simulink model "TV_2021"  (R2017b)
settings: Solver=VariableStepAuto  StartTime=0.0  StopTime=10.0  RelTol=1e-3
undefined symbols (not defined in the file): sigbuilder_block
libraries: simulink x6
(part 8 of 13)

== system TV_2021/Vehicle Dynamics Control 2018/Steering TV 2017 with TC/Constraints/current_limitation1/constants_saturator ==
  note: Saturamos con unos
      | valores máximos
      | preestablecidos
  allowed_current [%] : Inport
  max_discharge_current : Inport  Port=2
  max_regen_current : Inport  Port=3
  Constant : Constant  Value=0
  Gain2 : Gain  Gain=-1
  Saturation Dynamic : simulink/Discontinuities/Saturation Dynamic  OutMin=[]  OutMax=[]  OutDataTypeStr=Inherit: Same as second input  OutDataType=fixdt(1, 16)  OutScaling=2^-10  DoSatur=off
  Saturation Dynamic1 : simulink/Discontinuities/Saturation Dynamic  OutMin=[]  OutMax=[]  OutDataTypeStr=Inherit: Same as second input  OutDataType=fixdt(1, 16)  OutScaling=2^-10  DoSatur=off
  limited_discharge_actual : Outport  VectorParamsAs1DForOutWhenUnconnected=on
  limited_regen_actual : Outport  Port=2  VectorParamsAs1DForOutWhenUnconnected=on
  wires:
  max_regen_current/1 -> Saturation Dynamic1/1
  Constant/1 -> Saturation Dynamic/3, Saturation Dynamic1/3
  Gain2/1 -> Saturation Dynamic1/2
  Saturation Dynamic1/1 -> limited_regen_actual/1
  allowed_current [%]/1 -> Saturation Dynamic/2, Gain2/1
  Saturation Dynamic/1 -> limited_discharge_actual/1
  max_discharge_current/1 -> Saturation Dynamic/1

== system TV_2021/Vehicle Dynamics Control 2018/Steering TV 2017 with TC/Constraints/current_limitation1/temperature_rise_limitator ==
  note: initial_limitation es una constante para la reducción inicial (de 0 a 1, más bajo significa que cambia
      | menos, más alto la limitación
      | inicial es más bestia).
  note: saturamos de 1 a 0 por si acaso
  note: magia chunga para
      | que los números cuadren
  note: Se limita la corriente en proporción
      | al ratio entre la temperatura actual y 50ºC
  note: output 0 si está por
      | debajo de 50ºC, 1 si está
      | por encima
  max_cell_temp : Inport
  initial_limitation : Inport  Port=2
  Add1 : Sum  Inputs=-+
  Add2 : Sum  Inputs=-++
  Add3 : Sum  Inputs=+-
  Constant1 : Constant  Value=55
  Constant2 : Constant  Value=5
  Constant3 : Constant
  Divide : Product  Inputs=*/
  Product4 : Product
  Saturation1 : Saturate  UpperLimit=1  LowerLimit=0
  Scope2 : Scope
  Scope4 : Scope
  Temp higher than 50 : simulink/Logic and Bit Operations/Compare To Constant  relop=>=  const=50  OutDataTypeStr=boolean  ZeroCross=off
  allowed_current : Outport  VectorParamsAs1DForOutWhenUnconnected=on
  wires:
  Divide/1 -> Add3/1
  Constant3/1 -> Add2/3
  Constant1/1 -> Divide/1
  max_cell_temp/1 -> Add1/2, Scope4/1, Temp higher than 50/1
  Temp higher than 50/1 -> Add2/1, Product4/2
  Constant2/1 -> Add1/1
  Product4/1 -> Add2/2
  Add2/1 -> Scope2/1, Saturation1/1
  Add3/1 -> Product4/1
  Add1/1 -> Divide/2
  Saturation1/1 -> allowed_current/1
  initial_limitation/1 -> Add3/2

== system TV_2021/Vehicle Dynamics Control 2018/Steering TV 2017 with TC/Optimization SKF & CKF/Subsystem /CKF ==
  Derivative : Inport
  CKF_Initial : Inport  Port=2
  "CKF_prev " : Inport  Port=3
  Cte_CKF : Inport  Port=4
  Action Port : ActionPort
  If1 : If  IfExpression=u1 >= 900  ElseIfExpressions=u1 < 900  ShowElse=off
  Merge : Merge
  No spin : Subsystem  TreatAsAtomicUnit=on
  Saturation : Saturate  UpperLimit=1  LowerLimit=0.3
  "Spin " : Subsystem  TreatAsAtomicUnit=on
  "CKF_act " : Outport
  wires:
  Merge/1 -> Saturation/1
  "CKF_prev "/1 -> "Spin "/1(CKF_prev), No spin/2(CKF_prev)
  If1/1 -> "Spin "/Action
  Cte_CKF/1 -> "Spin "/3(Cte_CKF)
  "Spin "/1("CKF_act1 ") -> Merge/2
  Saturation/1 -> "CKF_act "/1
  CKF_Initial/1 -> "Spin "/2("CKF_Initial "), No spin/1(CKF_Initial)
  If1/2 -> No spin/Action
  No spin/1(CKF_act0) -> Merge/1
  Derivative/1 -> If1/1

== system TV_2021/Vehicle Dynamics Control 2018/Steering TV 2017 with TC/Optimization SKF & CKF/Subsystem /SKF ==
  Derivative : Inport
  "SKF_Initial " : Inport  Port=2
  SKF_prev : Inport  Port=3
  Cte_SKF : Inport  Port=4
  Action Port : ActionPort
  Display : Display
  Display1 : Display
  If : If  IfExpression=u1 >=900  ElseIfExpressions=u1 < 900  ShowElse=off
  Merge : Merge
  No spin : Subsystem  TreatAsAtomicUnit=on
  Saturation : Saturate  UpperLimit=1  LowerLimit=0.3
  Spin : Subsystem  TreatAsAtomicUnit=on
  SKF_act : Outport
  wires:
  Merge/1 -> Saturation/1
  Spin/1(SKF_act1) -> Merge/2
  "SKF_Initial "/1 -> Spin/1(SKF_Initial), No spin/1(SKF_Initial)
  No spin/1(SKF_act0) -> Merge/1
  If/2 -> No spin/Action
  SKF_prev/1 -> Display/1, Spin/2(SKF_prev), No spin/2(SKF_prev)
  Cte_SKF/1 -> Spin/3(Cte_SKF)
  Saturation/1 -> Display1/1, SKF_act/1
  If/1 -> Spin/Action
  Derivative/1 -> If/1

== system TV_2021/Vehicle Dynamics Control 2018/VDC 2018 Complete/Constraints/Acelerating and braking without Regenerative/Control de Potencia  ==
  Tq_RR : Inport
  Tq_RL : Inport  Port=2
  ReductionCte : Inport  Port=3
  Action Port : ActionPort
  Add : Sum  Inputs=+-
  Add1 : Sum  Inputs=+-
  Constant : Constant  Value=0
  Constant1 : Constant
  Product : Product
  Product1 : Product
  Tq_RR_out : Outport
  Tq_RL_out : Outport  Port=2
  Flag_Temperature : Outport  Port=3
  Flag_Power : Outport  Port=4
  wires:
  Tq_RR/1 -> Product/1, Add/1
  Tq_RL/1 -> Product1/1, Add1/1
  ReductionCte/1 -> Product/2, Product1/2
  Product1/1 -> Add1/2
  Product/1 -> Add/2
  Add1/1 -> Tq_RL_out/1
  Add/1 -> Tq_RR_out/1
  Constant1/1 -> Flag_Power/1
  Constant/1 -> Flag_Temperature/1

== system TV_2021/Vehicle Dynamics Control 2018/VDC 2018 Complete/Constraints/Acelerating and braking without Regenerative/Control de Temperatura ==
  Tq_RR : Inport
  Tq_RL : Inport  Port=2
  ReductionCte : Inport  Port=3
  Action Port : ActionPort
  Add : Sum  Inputs=+-
  Add1 : Sum  Inputs=+-
  Constant : Constant
  Constant1 : Constant  Value=0
  Product : Product
  Product1 : Product
  Tq_RR_out : Outport
  Tq_RL_out : Outport  Port=2
  Flag_Temperature : Outport  Port=3
  Flag_Power : Outport  Port=4
  wires:
  Add/1 -> Tq_RR_out/1
  Add1/1 -> Tq_RL_out/1
  Product/1 -> Add/2
  Product1/1 -> Add1/2
  ReductionCte/1 -> Product1/2, Product/2
  Tq_RL/1 -> Add1/1, Product1/1
  Tq_RR/1 -> Add/1, Product/1
  Constant1/1 -> Flag_Power/1
  Constant/1 -> Flag_Temperature/1

== system TV_2021/Vehicle Dynamics Control 2018/VDC 2018 Complete/Constraints/Acelerating and braking without Regenerative/If Action 1 ==
  Trans_max_dynamic : Inport
  Action Port : ActionPort
  Trans_limit : Outport
  wires:
  Trans_max_dynamic/1 -> Trans_limit/1

== system TV_2021/Vehicle Dynamics Control 2018/VDC 2018 Complete/Constraints/Acelerating and braking without Regenerative/If Action 2 ==
  "Trans_max_static " : Inport
  Action Port : ActionPort
  Trans_limit : Outport
  wires:
  "Trans_max_static "/1 -> Trans_limit/1

== system TV_2021/Vehicle Dynamics Control 2018/VDC 2018 Complete/Constraints/Acelerating and braking without Regenerative/Momentum Z scaled ==
  Tq_RR_Lim : Inport
  Tq_RL_Lim : Inport  Port=2
  Tq_RR_wc : Inport  Port=3
  Tq_RL_wc : Inport  Port=4
  Tq_diff : Inport  Port=5
  Display : Display
  Display1 : Display
  MATLAB Function : MATLAB Function  TreatAsAtomicUnit=on
  TQ_RR : Outport
  TQ_RL : Outport  Port=2
  wires:
  Tq_RL_Lim/1 -> MATLAB Function/2(tq_RL_lim)
  Tq_RR_Lim/1 -> MATLAB Function/1(tq_RR_lim)
  Tq_RR_wc/1 -> MATLAB Function/3(tq_RR_wc)
  Tq_RL_wc/1 -> MATLAB Function/4(tq_RL_wc)
  MATLAB Function/1(TQ_RR) -> Display/1, TQ_RR/1
  MATLAB Function/2(TQ_RL) -> Display1/1, TQ_RL/1
  Tq_diff/1 -> MATLAB Function/5(tq_diff)

== system TV_2021/Vehicle Dynamics Control 2018/VDC 2018 Complete/Constraints/Acelerating and braking without Regenerative/else ==
  Tq_RR : Inport
  Tq_RL : Inport  Port=2
  Action Port : ActionPort
  Constant : Constant  Value=0
  Constant1 : Constant  Value=0
  Tq_RR_out : Outport
  Tq_RL_out : Outport  Port=2
  Flag_Temperature : Outport  Port=3
  Flag_Power : Outport  Port=4
  wires:
  Tq_RR/1 -> Tq_RR_out/1
  Tq_RL/1 -> Tq_RL_out/1
  Constant1/1 -> Flag_Power/1
  Constant/1 -> Flag_Temperature/1

== system TV_2021/Vehicle Dynamics Control 2018/VDC 2018 Complete/Lateral Dynamics/Tire Longitudinal Force Difference/ Momentum_Z to Longitudinal Force Difference ==
  "\tMomentumZ [Nm]" : Inport
  RearTrackwidth [m] : Inport  Port=2
  Constant : Constant  Value=2
  Divide : Product  Inputs=*/
  Divide1 : Product  Inputs=*/
  Fx_diff [N] : Outport
  wires:
  Divide/1 -> Fx_diff [N]/1
  Divide1/1 -> Divide/2
  "\tMomentumZ [Nm]"/1 -> Divide/1
  Constant/1 -> Divide1/2
  RearTrackwidth [m]/1 -> Divide1/1

== system TV_2021/Vehicle Dynamics Control 2018/VDC 2018 Complete/Lateral Dynamics/Tire Longitudinal Force Difference/Momentum respect to Z-axis to correct the error ==
  Yaw_error_[º/s] : Inport
  Iz [kg/m^3] : Inport  Port=2
  Correction_Time [s] : Inport  Port=3
  Divide : Product  Inputs=*/
  Product : Product
  Momentum_Z [Nm] : Outport
  wires:
  Divide/1 -> Momentum_Z [Nm]/1
  Correction_Time [s]/1 -> Divide/2
  Product/1 -> Divide/1
  Yaw_error_[º/s]/1 -> Product/1
  Iz [kg/m^3]/1 -> Product/2

== system TV_2021/Vehicle Dynamics Control 2018/VDC 2018 Complete/Optimization SKF & CKF/Subsystem /CKF ==
  Derivative : Inport
  CKF_Initial : Inport  Port=2
  "CKF_prev " : Inport  Port=3
  Cte_CKF : Inport  Port=4
  Action Port : ActionPort
  If1 : If  IfExpression=u1 >= 900  ElseIfExpressions=u1 < 900  ShowElse=off
  Merge : Merge
  No spin : Subsystem  TreatAsAtomicUnit=on
  Saturation : Saturate  UpperLimit=1  LowerLimit=0.3
  "Spin " : Subsystem  TreatAsAtomicUnit=on
  "CKF_act " : Outport
  wires:
  Merge/1 -> Saturation/1
  "CKF_prev "/1 -> "Spin "/1(CKF_prev), No spin/2(CKF_prev)
  If1/1 -> "Spin "/Action
  Derivative/1 -> If1/1
  Cte_CKF/1 -> "Spin "/3(Cte_CKF)
  "Spin "/1("CKF_act1 ") -> Merge/2
  Saturation/1 -> "CKF_act "/1
  CKF_Initial/1 -> "Spin "/2("CKF_Initial "), No spin/1(CKF_Initial)
  If1/2 -> No spin/Action
  No spin/1(CKF_act0) -> Merge/1

== system TV_2021/Vehicle Dynamics Control 2018/VDC 2018 Complete/Optimization SKF & CKF/Subsystem /SKF ==
  Derivative : Inport
  "SKF_Initial " : Inport  Port=2
  SKF_prev : Inport  Port=3
  Cte_SKF : Inport  Port=4
  Action Port : ActionPort
  Display : Display
  If : If  IfExpression=u1 >=900  ElseIfExpressions=u1 < 900  ShowElse=off
  Merge : Merge
  No spin : Subsystem  TreatAsAtomicUnit=on
  Saturation : Saturate  UpperLimit=1  LowerLimit=0.3
  Spin : Subsystem  TreatAsAtomicUnit=on
  SKF_act : Outport
  wires:
  Merge/1 -> Saturation/1
  Derivative/1 -> If/1, Display/1
  Spin/1(SKF_act1) -> Merge/2
  "SKF_Initial "/1 -> Spin/1(SKF_Initial), No spin/1(SKF_Initial)
  No spin/1(SKF_act0) -> Merge/1
  If/2 -> No spin/Action
  SKF_prev/1 -> Spin/2(SKF_prev), No spin/2(SKF_prev)
  Cte_SKF/1 -> Spin/3(Cte_SKF)
  Saturation/1 -> SKF_act/1
  If/1 -> Spin/Action

== system TV_2021/Vehicle Dynamics Control 2018/VDC 2018 without Longitudinal/Constraints/Acelerating and braking without Regenerative/Control de Potencia 1 ==
  Tq_RR : Inport
  Tq_RL : Inport  Port=2
  ReductionCte : Inport  Port=3
  Action Port : ActionPort
  Add : Sum  Inputs=+-
  Add1 : Sum  Inputs=+-
  Product : Product
  Product1 : Product
  Tq_RR_out : Outport
  Tq_RL_out : Outport  Port=2
  wires:
  Tq_RR/1 -> Product/1, Add/1
  Tq_RL/1 -> Product1/1, Add1/1
  ReductionCte/1 -> Product/2, Product1/2
  Product1/1 -> Add1/2
  Product/1 -> Add/2
  Add1/1 -> Tq_RL_out/1
  Add/1 -> Tq_RR_out/1

== system TV_2021/Vehicle Dynamics Control 2018/VDC 2018 without Longitudinal/Constraints/Acelerating and braking without Regenerative/Control de Temperatura1 ==
  Tq_RR : Inport
  Tq_RL : Inport  Port=2
  ReductionCte : Inport  Port=3
  Action Port : ActionPort
  Add : Sum  Inputs=+-
  Add1 : Sum  Inputs=+-
  Product : Product
  Product1 : Product
  Tq_RR_out : Outport
  Tq_RL_out : Outport  Port=2
  wires:
  Product/1 -> Add/2
  Product1/1 -> Add1/2
  Add1/1 -> Tq_RL_out/1
  Tq_RR/1 -> Add/1, Product/1
  Tq_RL/1 -> Add1/1, Product1/1
  ReductionCte/1 -> Product1/2, Product/2
  Add/1 -> Tq_RR_out/1

== system TV_2021/Vehicle Dynamics Control 2018/VDC 2018 without Longitudinal/Constraints/Acelerating and braking without Regenerative/If Action 1 ==
  Trans_max_dynamic : Inport
  Action Port : ActionPort
  Trans_limit : Outport
  wires:
  Trans_max_dynamic/1 -> Trans_limit/1

== system TV_2021/Vehicle Dynamics Control 2018/VDC 2018 without Longitudinal/Constraints/Acelerating and braking without Regenerative/If Action 2 ==
  "Trans_max_static " : Inport
  Action Port : ActionPort
  Trans_limit : Outport
  wires:
  "Trans_max_static "/1 -> Trans_limit/1

== system TV_2021/Vehicle Dynamics Control 2018/VDC 2018 without Longitudinal/Constraints/Acelerating and braking without Regenerative/Momentum Z scaled ==
  Tq_RR_Lim : Inport
  Tq_RL_Lim : Inport  Port=2
  Tq_RR_wc : Inport  Port=3
  Tq_RL_wc : Inport  Port=4
  MATLAB Function : MATLAB Function  TreatAsAtomicUnit=on
  TQ_RR : Outport
  TQ_RL : Outport  Port=2
  wires:
  Tq_RL_Lim/1 -> MATLAB Function/2(tq_RL_lim)
  Tq_RR_Lim/1 -> MATLAB Function/1(tq_RR_lim)
  Tq_RR_wc/1 -> MATLAB Function/3(tq_RR_wc)
  Tq_RL_wc/1 -> MATLAB Function/4(tq_RL_wc)
  MATLAB Function/1(TQ_RR) -> TQ_RR/1
  MATLAB Function/2(TQ_RL) -> TQ_RL/1

== system TV_2021/Vehicle Dynamics Control 2018/VDC 2018 without Longitudinal/Constraints/Acelerating and braking without Regenerative/else1 ==
  Tq_RR : Inport
  Tq_RL : Inport  Port=2
  Action Port : ActionPort
  Tq_RR_out : Outport
  Tq_RL_out : Outport  Port=2
  wires:
  Tq_RR/1 -> Tq_RR_out/1
  Tq_RL/1 -> Tq_RL_out/1

== system TV_2021/Vehicle Dynamics Control 2018/VDC 2018 without Longitudinal/Optimization SKF & CKF/Subsystem /CKF ==
  Derivative : Inport
  CKF_Initial : Inport  Port=2
  "CKF_prev " : Inport  Port=3
  Cte_CKF : Inport  Port=4
  If1 : If  IfExpression=u1 >= 900  ElseIfExpressions=u1 < 900  ShowElse=off
  Merge : Merge
  No spin : Subsystem  TreatAsAtomicUnit=on
  Saturation : Saturate  UpperLimit=1  LowerLimit=0.3
  "Spin " : Subsystem  TreatAsAtomicUnit=on
  "CKF_act " : Outport
  wires:
  Merge/1 -> Saturation/1
  "CKF_prev "/1 -> "Spin "/1(CKF_prev), No spin/2(CKF_prev)
  Derivative/1 -> If1/1
  Cte_CKF/1 -> "Spin "/3(Cte_CKF)
  "Spin "/1("CKF_act1 ") -> Merge/2
  Saturation/1 -> "CKF_act "/1
  CKF_Initial/1 -> "Spin "/2("CKF_Initial "), No spin/1(CKF_Initial)
  If1/2 -> No spin/Action
  No spin/1(CKF_act0) -> Merge/1
  If1/1 -> "Spin "/Action

== system TV_2021/If Action Subsystem1/Steering TV 2017 with TC/Optimization SKF & CKF/Subsystem /CKF/No spin ==
  CKF_Initial : Inport
  CKF_prev : Inport  Port=2
  Action Port : ActionPort
  MATLAB Function : MATLAB Function  TreatAsAtomicUnit=on
  Switch : Switch  Criteria=u2 > Threshold
  CKF_act0 : Outport
  wires:
  CKF_Initial/1 -> Switch/3, MATLAB Function/2(CKF_Initial)
  MATLAB Function/1(CKF_act0) -> CKF_act0/1
  CKF_prev/1 -> Switch/1, Switch/2
  Switch/1 -> MATLAB Function/1(CKF_prev)

== system TV_2021/If Action Subsystem1/Steering TV 2017 with TC/Optimization SKF & CKF/Subsystem /CKF/Spin  ==
  CKF_prev : Inport
  "CKF_Initial " : Inport  Port=2
  Cte_CKF : Inport  Port=3
  Action Port : ActionPort
  Constant : Constant
  MATLAB Function : MATLAB Function  TreatAsAtomicUnit=on
  Product : Product
  Switch : Switch  Criteria=u2 > Threshold  Threshold=0.9
  "CKF_act1 " : Outport
  wires:
  CKF_prev/1 -> Product/1
  MATLAB Function/1(CKF_act1) -> "CKF_act1 "/1
  Product/1 -> MATLAB Function/2(CKF_prev)
  "CKF_Initial "/1 -> MATLAB Function/1(CKF_Initial)
  Cte_CKF/1 -> Switch/2, Switch/1
  Constant/1 -> Switch/3
  Switch/1 -> Product/2

== system TV_2021/If Action Subsystem1/Steering TV 2017 with TC/Optimization SKF & CKF/Subsystem /SKF/No spin ==
  SKF_Initial : Inport
  SKF_prev : Inport  Port=2
  Action Port : ActionPort
  MATLAB Function : MATLAB Function  TreatAsAtomicUnit=on
  Switch : Switch  Criteria=u2 > Threshold
  SKF_act0 : Outport
  wires:
  SKF_Initial/1 -> MATLAB Function/2(SKF_Initial), Switch/3
  MATLAB Function/1(SKF_act0) -> SKF_act0/1
  SKF_prev/1 -> Switch/1, Switch/2
  Switch/1 -> MATLAB Function/1(SKF_prev)

== system TV_2021/If Action Subsystem1/Steering TV 2017 with TC/Optimization SKF & CKF/Subsystem /SKF/Spin ==
  SKF_Initial : Inport
  SKF_prev : Inport  Port=2
  Cte_SKF : Inport  Port=3
  Action Port : ActionPort
  Constant : Constant
  MATLAB Function : MATLAB Function  TreatAsAtomicUnit=on
  Product : Product
  Switch : Switch  Criteria=u2 > Threshold  Threshold=0.9
  SKF_act1 : Outport
  wires:
  SKF_Initial/1 -> MATLAB Function/1(SKF_Initial)
  Product/1 -> MATLAB Function/2(SKF_prev)
  MATLAB Function/1(SKF_act1) -> SKF_act1/1
  SKF_prev/1 -> Product/1
  Switch/1 -> Product/2
  Cte_SKF/1 -> Switch/2, Switch/1
  Constant/1 -> Switch/3

== system TV_2021/If Action Subsystem1/VDC 2018 Complete/Optimization SKF & CKF/Subsystem /CKF/No spin ==
  CKF_Initial : Inport
  CKF_prev : Inport  Port=2
  Action Port : ActionPort
  MATLAB Function : MATLAB Function  TreatAsAtomicUnit=on
  Switch : Switch  Criteria=u2 > Threshold
  CKF_act0 : Outport
  wires:
  CKF_Initial/1 -> Switch/3, MATLAB Function/2(CKF_Initial)
  MATLAB Function/1(CKF_act0) -> CKF_act0/1
  CKF_prev/1 -> Switch/1, Switch/2
  Switch/1 -> MATLAB Function/1(CKF_prev)

== system TV_2021/If Action Subsystem1/VDC 2018 Complete/Optimization SKF & CKF/Subsystem /CKF/Spin  ==
  CKF_prev : Inport
  "CKF_Initial " : Inport  Port=2
  Cte_CKF : Inport  Port=3
  Action Port : ActionPort
  Constant : Constant
  MATLAB Function : MATLAB Function  TreatAsAtomicUnit=on
  Product : Product
  Switch : Switch  Criteria=u2 > Threshold  Threshold=0.9
  "CKF_act1 " : Outport
  wires:
  CKF_prev/1 -> Product/1
  MATLAB Function/1(CKF_act1) -> "CKF_act1 "/1
  Product/1 -> MATLAB Function/2(CKF_prev)
  "CKF_Initial "/1 -> MATLAB Function/1(CKF_Initial)
  Cte_CKF/1 -> Switch/2, Switch/1
  Constant/1 -> Switch/3
  Switch/1 -> Product/2

== system TV_2021/If Action Subsystem1/VDC 2018 Complete/Optimization SKF & CKF/Subsystem /SKF/No spin ==
  SKF_Initial : Inport
  SKF_prev : Inport  Port=2
  Action Port : ActionPort
  MATLAB Function : MATLAB Function  TreatAsAtomicUnit=on
  Switch : Switch  Criteria=u2 > Threshold
  SKF_act0 : Outport
  wires:
  SKF_Initial/1 -> MATLAB Function/2(SKF_Initial), Switch/3
  MATLAB Function/1(SKF_act0) -> SKF_act0/1
  SKF_prev/1 -> Switch/1, Switch/2
  Switch/1 -> MATLAB Function/1(SKF_prev)

== system TV_2021/If Action Subsystem1/VDC 2018 Complete/Optimization SKF & CKF/Subsystem /SKF/Spin ==
  SKF_Initial : Inport
  SKF_prev : Inport  Port=2
  Cte_SKF : Inport  Port=3
  Action Port : ActionPort
  Constant : Constant
  MATLAB Function : MATLAB Function  TreatAsAtomicUnit=on
  Product : Product
  Switch : Switch  Criteria=u2 > Threshold  Threshold=0.9
  SKF_act1 : Outport
  wires:
  SKF_Initial/1 -> MATLAB Function/1(SKF_Initial)
  Product/1 -> MATLAB Function/2(SKF_prev)
  MATLAB Function/1(SKF_act1) -> SKF_act1/1
  SKF_prev/1 -> Product/1
  Switch/1 -> Product/2
  Cte_SKF/1 -> Switch/2, Switch/1
  Constant/1 -> Switch/3

== system TV_2021/If Action Subsystem1/VDC 2018 without Longitudinal/Optimization SKF & CKF/Subsystem /CKF/No spin ==
  CKF_Initial : Inport
  CKF_prev : Inport  Port=2
  Action Port : ActionPort
  MATLAB Function : MATLAB Function  TreatAsAtomicUnit=on
  Switch : Switch  Criteria=u2 > Threshold
  CKF_act0 : Outport
  wires:
  CKF_Initial/1 -> Switch/3, MATLAB Function/2(CKF_Initial)
  MATLAB Function/1(CKF_act0) -> CKF_act0/1
  CKF_prev/1 -> Switch/1, Switch/2
  Switch/1 -> MATLAB Function/1(CKF_prev)

== system TV_2021/If Action Subsystem1/VDC 2018 without Longitudinal/Optimization SKF & CKF/Subsystem /CKF/Spin  ==
  CKF_prev : Inport
  "CKF_Initial " : Inport  Port=2
  Cte_CKF : Inport  Port=3
  Action Port : ActionPort
  Constant : Constant
  MATLAB Function : MATLAB Function  TreatAsAtomicUnit=on
  Product : Product
  Switch : Switch  Criteria=u2 > Threshold  Threshold=0.9
  "CKF_act1 " : Outport
  wires:
  CKF_prev/1 -> Product/1
  MATLAB Function/1(CKF_act1) -> "CKF_act1 "/1
  Product/1 -> MATLAB Function/2(CKF_prev)
  "CKF_Initial "/1 -> MATLAB Function/1(CKF_Initial)
  Cte_CKF/1 -> Switch/2, Switch/1
  Constant/1 -> Switch/3
  Switch/1 -> Product/2

== system TV_2021/Vehicle Dynamics Control 1/Steering TV 2017 with TC/Optimization SKF & CKF/Subsystem /CKF/No spin ==
  CKF_Initial : Inport
  CKF_prev : Inport  Port=2
  Action Port : ActionPort
  Display : Display
  Display1 : Display
  MATLAB Function : MATLAB Function  TreatAsAtomicUnit=on
  Switch : Switch  Criteria=u2 > Threshold
  CKF_act0 : Outport
  wires:
  Switch/1 -> MATLAB Function/1(CKF_prev), Display/1
  CKF_prev/1 -> Switch/2, Switch/1
  MATLAB Function/1(CKF_act0) -> Display1/1, CKF_act0/1
  CKF_Initial/1 -> MATLAB Function/2(CKF_Initial), Switch/3

== system TV_2021/Vehicle Dynamics Control 1/Steering TV 2017 with TC/Optimization SKF & CKF/Subsystem /CKF/Spin  ==
  CKF_prev : Inport
  "CKF_Initial " : Inport  Port=2
  Cte_CKF : Inport  Port=3
  Action Port : ActionPort
  Constant : Constant
  Display : Display
  Display1 : Display
  Display2 : Display
  MATLAB Function : MATLAB Function  TreatAsAtomicUnit=on
  Product : Product
  Switch : Switch  Criteria=u2 > Threshold  Threshold=0.9
  "CKF_act1 " : Outport
  wires:
  Switch/1 -> Product/2
  Constant/1 -> Switch/3
  Cte_CKF/1 -> Switch/1, Switch/2
  "CKF_Initial "/1 -> MATLAB Function/1(CKF_Initial)
  Product/1 -> MATLAB Function/2(CKF_prev), Display/1
  MATLAB Function/1(CKF_act1) -> Display1/1, "CKF_act1 "/1
  CKF_prev/1 -> Display2/1, Product/1

== system TV_2021/Vehicle Dynamics Control 1/Steering TV 2017 with TC/Optimization SKF & CKF/Subsystem /SKF/No spin ==
  SKF_Initial : Inport
  SKF_prev : Inport  Port=2
  Action Port : ActionPort
  Display : Display
  Display1 : Display
  MATLAB Function : MATLAB Function  TreatAsAtomicUnit=on
  Switch : Switch  Criteria=u2 > Threshold
  SKF_act0 : Outport
  wires:
  SKF_prev/1 -> Switch/2, Switch/1, Display1/1
  Switch/1 -> MATLAB Function/1(SKF_prev)
  MATLAB Function/1(SKF_act0) -> SKF_act0/1, Display/1
  SKF_Initial/1 -> Switch/3, MATLAB Function/2(SKF_Initial)

== system TV_2021/Vehicle Dynamics Control 1/Steering TV 2017 with TC/Optimization SKF & CKF/Subsystem /SKF/Spin ==
  SKF_Initial : Inport
  SKF_prev : Inport  Port=2
  Cte_SKF : Inport  Port=3
  Action Port : ActionPort
  Constant : Constant
  Display{,1..4} (5 alike) : Display
  MATLAB Function : MATLAB Function  TreatAsAtomicUnit=on
  Product : Product
  Switch : Switch  Criteria=u2 > Threshold  Threshold=0.9
  SKF_act1 : Outport
  wires:
  Constant/1 -> Switch/3
  Cte_SKF/1 -> Switch/1, Switch/2
  Switch/1 -> Product/2, Display4/1
  SKF_prev/1 -> Product/1, Display3/1
  MATLAB Function/1(SKF_act1) -> Display2/1, SKF_act1/1
  Product/1 -> MATLAB Function/2(SKF_prev), Display1/1
  SKF_Initial/1 -> MATLAB Function/1(SKF_Initial), Display/1

== system TV_2021/Vehicle Dynamics Control 1/VDC 2018 Complete/Optimization SKF & CKF/Subsystem /CKF/No spin ==
  CKF_Initial : Inport
  CKF_prev : Inport  Port=2
  Action Port : ActionPort
  MATLAB Function : MATLAB Function  TreatAsAtomicUnit=on
  Switch : Switch  Criteria=u2 > Threshold
  CKF_act0 : Outport
  wires:
  Switch/1 -> MATLAB Function/1(CKF_prev)
  CKF_prev/1 -> Switch/2, Switch/1
  MATLAB Function/1(CKF_act0) -> CKF_act0/1
  CKF_Initial/1 -> MATLAB Function/2(CKF_Initial), Switch/3

== system TV_2021/Vehicle Dynamics Control 1/VDC 2018 Complete/Optimization SKF & CKF/Subsystem /CKF/Spin  ==
  CKF_prev : Inport
  "CKF_Initial " : Inport  Port=2
  Cte_CKF : Inport  Port=3
  Action Port : ActionPort
  Constant : Constant
  MATLAB Function : MATLAB Function  TreatAsAtomicUnit=on
  Product : Product
  Switch : Switch  Criteria=u2 > Threshold  Threshold=0.9
  "CKF_act1 " : Outport
  wires:
  Switch/1 -> Product/2
  Constant/1 -> Switch/3
  Cte_CKF/1 -> Switch/1, Switch/2
  "CKF_Initial "/1 -> MATLAB Function/1(CKF_Initial)
  Product/1 -> MATLAB Function/2(CKF_prev)
  MATLAB Function/1(CKF_act1) -> "CKF_act1 "/1
  CKF_prev/1 -> Product/1

== system TV_2021/Vehicle Dynamics Control 1/VDC 2018 Complete/Optimization SKF & CKF/Subsystem /SKF/No spin ==
  SKF_Initial : Inport
  SKF_prev : Inport  Port=2
  Action Port : ActionPort
  MATLAB Function : MATLAB Function  TreatAsAtomicUnit=on
  Switch : Switch  Criteria=u2 > Threshold
  SKF_act0 : Outport
  wires:
  Switch/1 -> MATLAB Function/1(SKF_prev)
  SKF_prev/1 -> Switch/2, Switch/1
  MATLAB Function/1(SKF_act0) -> SKF_act0/1
  SKF_Initial/1 -> Switch/3, MATLAB Function/2(SKF_Initial)

== system TV_2021/Vehicle Dynamics Control 1/VDC 2018 Complete/Optimization SKF & CKF/Subsystem /SKF/Spin ==
  SKF_Initial : Inport
  SKF_prev : Inport  Port=2
  Cte_SKF : Inport  Port=3
  Action Port : ActionPort
  Constant : Constant
  MATLAB Function : MATLAB Function  TreatAsAtomicUnit=on
  Product : Product
  Switch : Switch  Criteria=u2 > Threshold  Threshold=0.9
  SKF_act1 : Outport
  wires:
  Constant/1 -> Switch/3
  Cte_SKF/1 -> Switch/1, Switch/2
  Switch/1 -> Product/2
  SKF_prev/1 -> Product/1
  MATLAB Function/1(SKF_act1) -> SKF_act1/1
  Product/1 -> MATLAB Function/2(SKF_prev)
  SKF_Initial/1 -> MATLAB Function/1(SKF_Initial)

== system TV_2021/Vehicle Dynamics Control 1/VDC 2018 without Longitudinal/Optimization SKF & CKF/Subsystem /CKF/No spin ==
  CKF_Initial : Inport
  CKF_prev : Inport  Port=2
  Action Port : ActionPort
  MATLAB Function : MATLAB Function  TreatAsAtomicUnit=on
  Switch : Switch  Criteria=u2 > Threshold
  CKF_act0 : Outport
  wires:
  Switch/1 -> MATLAB Function/1(CKF_prev)
  CKF_prev/1 -> Switch/2, Switch/1
  MATLAB Function/1(CKF_act0) -> CKF_act0/1
  CKF_Initial/1 -> MATLAB Function/2(CKF_Initial), Switch/3

== system TV_2021/Vehicle Dynamics Control 1/VDC 2018 without Longitudinal/Optimization SKF & CKF/Subsystem /CKF/Spin  ==
  CKF_prev : Inport
  "CKF_Initial " : Inport  Port=2
  Cte_CKF : Inport  Port=3
  Action Port : ActionPort
  Constant : Constant
  MATLAB Function : MATLAB Function  TreatAsAtomicUnit=on
  Product : Product
  Switch : Switch  Criteria=u2 > Threshold  Threshold=0.9
  "CKF_act1 " : Outport
  wires:
  Switch/1 -> Product/2
  Constant/1 -> Switch/3
  Cte_CKF/1 -> Switch/1, Switch/2
  "CKF_Initial "/1 -> MATLAB Function/1(CKF_Initial)
  Product/1 -> MATLAB Function/2(CKF_prev)
  MATLAB Function/1(CKF_act1) -> "CKF_act1 "/1
  CKF_prev/1 -> Product/1

== system TV_2021/Vehicle Dynamics Control 2018/Steering TV 2017 with TC/Optimization SKF & CKF/Subsystem /CKF/No spin ==
  CKF_Initial : Inport
  CKF_prev : Inport  Port=2
  Action Port : ActionPort
  Display : Display
  Display1 : Display
  MATLAB Function : MATLAB Function  TreatAsAtomicUnit=on
  Switch : Switch  Criteria=u2 > Threshold
  CKF_act0 : Outport
  wires:
  CKF_Initial/1 -> Switch/3, MATLAB Function/2(CKF_Initial)
  MATLAB Function/1(CKF_act0) -> CKF_act0/1, Display1/1
  CKF_prev/1 -> Switch/1, Switch/2
  Switch/1 -> Display/1, MATLAB Function/1(CKF_prev)

== system TV_2021/Vehicle Dynamics Control 2018/Steering TV 2017 with TC/Optimization SKF & CKF/Subsystem /CKF/Spin  ==
  CKF_prev : Inport
  "CKF_Initial " : Inport  Port=2
  Cte_CKF : Inport  Port=3
  Action Port : ActionPort
  Constant : Constant
  Display : Display
  Display1 : Display
  Display2 : Display
  MATLAB Function : MATLAB Function  TreatAsAtomicUnit=on
  Product : Product
  Switch : Switch  Criteria=u2 > Threshold  Threshold=0.9
  "CKF_act1 " : Outport
  wires:
  CKF_prev/1 -> Product/1, Display2/1
  MATLAB Function/1(CKF_act1) -> "CKF_act1 "/1, Display1/1
  Product/1 -> Display/1, MATLAB Function/2(CKF_prev)
  "CKF_Initial "/1 -> MATLAB Function/1(CKF_Initial)
  Cte_CKF/1 -> Switch/2, Switch/1
  Constant/1 -> Switch/3
  Switch/1 -> Product/2

== system TV_2021/Vehicle Dynamics Control 2018/Steering TV 2017 with TC/Optimization SKF & CKF/Subsystem /SKF/No spin ==
  SKF_Initial : Inport
  SKF_prev : Inport  Port=2
  Action Port : ActionPort
  Display : Display
  Display1 : Display
  MATLAB Function : MATLAB Function  TreatAsAtomicUnit=on
  Switch : Switch  Criteria=u2 > Threshold
  SKF_act0 : Outport
  wires:
  SKF_Initial/1 -> MATLAB Function/2(SKF_Initial), Switch/3
  MATLAB Function/1(SKF_act0) -> Display/1, SKF_act0/1
  Switch/1 -> MATLAB Function/1(SKF_prev)
  SKF_prev/1 -> Display1/1, Switch/1, Switch/2

== system TV_2021/Vehicle Dynamics Control 2018/Steering TV 2017 with TC/Optimization SKF & CKF/Subsystem /SKF/Spin ==
  SKF_Initial : Inport
  SKF_prev : Inport  Port=2
  Cte_SKF : Inport  Port=3
  Action Port : ActionPort
  Constant : Constant
  Display{,1..4} (5 alike) : Display
  MATLAB Function : MATLAB Function  TreatAsAtomicUnit=on
  Product : Product
  Switch : Switch  Criteria=u2 > Threshold  Threshold=0.9
  SKF_act1 : Outport
  wires:
  SKF_Initial/1 -> Display/1, MATLAB Function/1(SKF_Initial)
  Product/1 -> Display1/1, MATLAB Function/2(SKF_prev)
  MATLAB Function/1(SKF_act1) -> SKF_act1/1, Display2/1
  SKF_prev/1 -> Display3/1, Product/1
  Switch/1 -> Display4/1, Product/2
  Cte_SKF/1 -> Switch/2, Switch/1
  Constant/1 -> Switch/3

== system TV_2021/Vehicle Dynamics Control 2018/VDC 2018 Complete/Optimization SKF & CKF/Subsystem /CKF/No spin ==
  CKF_Initial : Inport
  CKF_prev : Inport  Port=2
  Action Port : ActionPort
  MATLAB Function : MATLAB Function  TreatAsAtomicUnit=on
  Switch : Switch  Criteria=u2 > Threshold
  CKF_act0 : Outport
  wires:
  CKF_Initial/1 -> Switch/3, MATLAB Function/2(CKF_Initial)
  MATLAB Function/1(CKF_act0) -> CKF_act0/1
  CKF_prev/1 -> Switch/1, Switch/2
  Switch/1 -> MATLAB Function/1(CKF_prev)

== system TV_2021/Vehicle Dynamics Control 2018/VDC 2018 Complete/Optimization SKF & CKF/Subsystem /CKF/Spin  ==
  CKF_prev : Inport
  "CKF_Initial " : Inport  Port=2
  Cte_CKF : Inport  Port=3
  Action Port : ActionPort
  Constant : Constant
  MATLAB Function : MATLAB Function  TreatAsAtomicUnit=on
  Product : Product
  Switch : Switch  Criteria=u2 > Threshold  Threshold=0.9
  "CKF_act1 " : Outport
  wires:
  CKF_prev/1 -> Product/1
  MATLAB Function/1(CKF_act1) -> "CKF_act1 "/1
  Product/1 -> MATLAB Function/2(CKF_prev)
  "CKF_Initial "/1 -> MATLAB Function/1(CKF_Initial)
  Cte_CKF/1 -> Switch/2, Switch/1
  Constant/1 -> Switch/3
  Switch/1 -> Product/2

== system TV_2021/Vehicle Dynamics Control 2018/VDC 2018 Complete/Optimization SKF & CKF/Subsystem /SKF/No spin ==
  SKF_Initial : Inport
  SKF_prev : Inport  Port=2
  Action Port : ActionPort
  MATLAB Function : MATLAB Function  TreatAsAtomicUnit=on
  Switch : Switch  Criteria=u2 > Threshold
  SKF_act0 : Outport
  wires:
  SKF_Initial/1 -> MATLAB Function/2(SKF_Initial), Switch/3
  MATLAB Function/1(SKF_act0) -> SKF_act0/1
  SKF_prev/1 -> Switch/1, Switch/2
  Switch/1 -> MATLAB Function/1(SKF_prev)

== system TV_2021/Vehicle Dynamics Control 2018/VDC 2018 Complete/Optimization SKF & CKF/Subsystem /SKF/Spin ==
  SKF_Initial : Inport
  SKF_prev : Inport  Port=2
  Cte_SKF : Inport  Port=3
  Action Port : ActionPort
  Constant : Constant
  MATLAB Function : MATLAB Function  TreatAsAtomicUnit=on
  Product : Product
  Switch : Switch  Criteria=u2 > Threshold  Threshold=0.9
  SKF_act1 : Outport
  wires:
  SKF_Initial/1 -> MATLAB Function/1(SKF_Initial)
  Product/1 -> MATLAB Function/2(SKF_prev)
  MATLAB Function/1(SKF_act1) -> SKF_act1/1
  SKF_prev/1 -> Product/1
  Switch/1 -> Product/2
  Cte_SKF/1 -> Switch/2, Switch/1
  Constant/1 -> Switch/3

== system TV_2021/Vehicle Dynamics Control 2018/VDC 2018 without Longitudinal/Optimization SKF & CKF/Subsystem /CKF/No spin ==
  CKF_Initial : Inport
  CKF_prev : Inport  Port=2
  Action Port : ActionPort
  MATLAB Function : MATLAB Function  TreatAsAtomicUnit=on
  Switch : Switch  Criteria=u2 > Threshold
  CKF_act0 : Outport
  wires:
  CKF_Initial/1 -> Switch/3, MATLAB Function/2(CKF_Initial)
  MATLAB Function/1(CKF_act0) -> CKF_act0/1
  CKF_prev/1 -> Switch/1, Switch/2
  Switch/1 -> MATLAB Function/1(CKF_prev)

== system TV_2021/Vehicle Dynamics Control 2018/VDC 2018 without Longitudinal/Optimization SKF & CKF/Subsystem /CKF/Spin  ==
  CKF_prev : Inport
  "CKF_Initial " : Inport  Port=2
  Cte_CKF : Inport  Port=3
  Action Port : ActionPort
  Constant : Constant
  MATLAB Function : MATLAB Function  TreatAsAtomicUnit=on
  Product : Product
  Switch : Switch  Criteria=u2 > Threshold  Threshold=0.9
  "CKF_act1 " : Outport
  wires:
  CKF_prev/1 -> Product/1
  MATLAB Function/1(CKF_act1) -> "CKF_act1 "/1
  Product/1 -> MATLAB Function/2(CKF_prev)
  "CKF_Initial "/1 -> MATLAB Function/1(CKF_Initial)
  Cte_CKF/1 -> Switch/2, Switch/1
  Constant/1 -> Switch/3
  Switch/1 -> Product/2

== matlab function TV_2021/Vehicle Dynamics Control 2018/VDC 2018 Complete/Constraints/Acelerating and braking without Regenerative/MATLAB Function ==
  data: diff_wc input; diff_lim output; diff_max input
function diff_lim = fcn(diff_wc,diff_max)

if diff_wc < -diff_max
    diff_lim = -diff_max;
elseif diff_wc > diff_max
    diff_lim = diff_max;
else
    diff_lim = diff_wc;
end
